simulink model "iq"  (R2021a)
settings: Solver=VariableStepAuto  StartTime=0.0  StopTime=0.2  FixedStep=1/150000  MaxStep=1e-6
undefined symbols (not defined in the file): in, ou
libraries: neural x55, spsMosfetLib x12, simulink x5, pid_lib x3, spsFirstOrderFilterLib x2, spsPermanentMagnetSynchronousMachineLib x2, spsCurrentMeasurementLib x2, spsDCVoltageSourceLib x2, spsThreePhaseVIMeasurementLib x2, spsabctoAlphaBetaZeroLib x2, spsabctodq0Lib x2, spsSVPWMGenerator2LevelLib x1
(part 3 of 5)

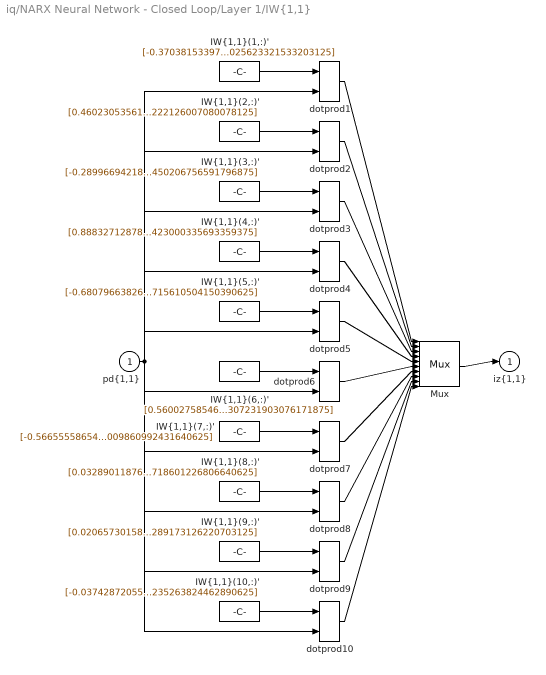
== system iq/NARX Neural Network - Closed Loop/Layer 1/IW{1,1} ==
  "pd{1,1}" : Inport  PortDimensions=40  SampleTime=1e-05
      mask Display: e = 0.06;c1 = [120 230 180]/255;c2 = ([120 230 180]+0)/(256+128);c3 = ([120 230 180]+128)/(256+128);patch([0 1 1 0],[0 0 1 1],c1);patch([0 1 1 1-e 1-e 0+e],[0 0 1 1-e 0+e 0+e],c2);patch([0 0 1 1-e 0+e 0+e],[0 1 1 1-e 1-e 0+e],c3);plot([0 1 1 0 0],[0 0 1 1 0]);
  "IW{1,1}(1,:)'" : Constant  Value=[-0.370381533971269993887887039818451739847660064697265625;-0.60836575089238376090605697754654102027416229248046875;-0.409154141847963559452949766637175343930721282958984375;-0.41099431863818447485670048990868963301181793212890625;0.582923557528958635742810656665824353694915771484375;0.48663433989662652212615512326010502874851226806640625;-0.36467940418610844677260729440604336559772491455078125;-0.357974175848268572064370118823717348277568817138671875;-0.05688146982302262621988830915142898447811603546142578125;0.27270848568918271137562214789795689284801483154296875;-0.278331288705670865102348443542723543941974639892578125;-0.297309238840328504682730681452085264027118682861328125;0.01329069212345795371332801693142755539156496524810791015625;0.147003708510372421702783185537555254995822906494140625;-0.18739990347048396390761126895085908472537994384765625;-0.2149201060465101564833645397811778821051120758056640625;-0.0917872157463859028592167987881111912429332733154296875;0.0035005746246020616983807283162377643748186528682708740234375;-0.08414655753051160369526684235097491182386875152587890625;-0.11492868974622892641601623608949012123048305511474609375;-0.06482294244093385338079116309017990715801715850830078125;-0.019538025462217778471796236772206611931324005126953125;0.0219420954523434526273195643852886860258877277374267578125;-0.000970026128533838329949523515693954323069192469120025634765625;0.1843367033017555833840361856346135027706623077392578125;0.130725146693732197089587998561910353600978851318359375;0.1154576707265280166581078447052277624607086181640625;0.12260015593334148975568353989729075692594051361083984375;-0.01254060663158583326104444921611502650193870067596435546875;0.10900370676490478416553742135874927043914794921875;0.222478076142917646773611295429873280227184295654296875;0.25070616152984681601623151436797343194484710693359375;-0.018515784184349119712020836914234678260982036590576171875;0.1284041153197590101608938084609690122306346893310546875;0.3337859120951376379338171318522654473781585693359375;0.383812488121198780444132125921896658837795257568359375;0.0961455234077264464520595765861799009144306182861328125;0.0307125609366359804408563860533831757493317127227783203125;0.446930741411597498569108211086131632328033447265625;0.5295339428349887800351325495284982025623321533203125]
      mask Display: e = 0.06;c1 = [120 150 230]/255;c2 = ([120 150 230]+0)/383;c3 = ([120 150 230]+128)/383;patch([0 1 1 0],[0 0 1 1],c1);patch([0 1 1 1-e 1-e 0+e],[0 0 1 1-e 0+e 0+e],c2);patch([0 0 1 1-e 0+e 0+e],[0 1 1 1-e 1-e 0+e],c3);plot([0 1 1 0 0],[0 0 1 1 0]);disp('Weights');
  "IW{1,1}(10,:)'" : Constant  Value=[-0.0374287205513150755820106496685184538364410400390625;0.70434564124573639798398971834103576838970184326171875;0.7522702909022649375714308916940353810787200927734375;-0.01261093693687474932840775210252104443497955799102783203125;-0.16170253340786666651496261692955158650875091552734375;-0.474734846451803138567271389547386206686496734619140625;0.58439215063359239987761384327313862740993499755859375;-0.023452774793525442420527582498834817670285701751708984375;-0.051992213555422862880650569650242687202990055084228515625;-0.402207742424022074434475371162989176809787750244140625;0.42010037354778428930757172565790824592113494873046875;-0.0264409316169393060480530266431742347776889801025390625;-0.1008865583285370182142770545397070236504077911376953125;-0.07089440261923037056579488535135169513523578643798828125;0.25870929446493751147073680840549059212207794189453125;-0.03930245328464300469395453774268389679491519927978515625;-0.15201157241618290516527167710592038929462432861328125;0.0679762667751536431293146733878529630601406097412109375;0.10520308939002430415055044932159944437444210052490234375;-0.0519526257417461945209424811764620244503021240234375;0.112774459926445358437518962091417051851749420166015625;0.12084052506689790806859718941268511116504669189453125;-0.052530615658511088661430932233997737057507038116455078125;-0.05120989834213336699964003173590754158794879913330078125;-0.12787210870842657950419152257381938397884368896484375;-0.078859476464717970234374888605088926851749420166015625;-0.182759134971150760673452850824105553328990936279296875;-0.037707706527031710497244176849562791176140308380126953125;-0.1480260727570686107856801072557573206722736358642578125;-0.0898293705578910028908268259328906424343585968017578125;-0.30135726108675431333949745749123394489288330078125;-0.0159454355043238717171139029460391611792147159576416015625;-0.1729662225865224167709044422736042179167270660400390625;-0.1563023964206002036636533603086718358099460601806640625;-0.405696085122499605635226771482848562300205230712890625;0.015662463760211853269765924778766930103302001953125;-0.06488524778837374828999173814736423082649707794189453125;0.08054078478975036647913299248102703131735324859619140625;-0.51152581330454705010879479232244193553924560546875;0.04378511372238913512688895934843458235263824462890625]
      mask Display: e = 0.06;c1 = [120 150 230]/255;c2 = ([120 150 230]+0)/383;c3 = ([120 150 230]+128)/383;patch([0 1 1 0],[0 0 1 1],c1);patch([0 1 1 1-e 1-e 0+e],[0 0 1 1-e 0+e 0+e],c2);patch([0 0 1 1-e 0+e 0+e],[0 1 1 1-e 1-e 0+e],c3);plot([0 1 1 0 0],[0 0 1 1 0]);disp('Weights');
  "IW{1,1}(2,:)'" : Constant  Value=[0.460230535615414770855835513430065475404262542724609375;-0.77110343400352954201792954336269758641719818115234375;-0.568625192561625691922699843416921794414520263671875;-0.919509208600904681674137464142404496669769287109375;-0.39640401774455680250497380257002077996730804443359375;0.7419835566523342862410572706721723079681396484375;-0.381755551532974302109124664639239199459552764892578125;-0.7087456477505529317539867406594567000865936279296875;-0.17918201870643091222490284053492359817028045654296875;0.267758509192989324620981506086536683142185211181640625;-0.2141562734063510997639667721159639768302440643310546875;-0.485468237640969968449411453548236750066280364990234375;0.073912236857971047587767543518566526472568511962890625;0.26681110876441505030953749155742116272449493408203125;-0.080785181060193222979393112836987711489200592041015625;-0.2730384489657227131687022847472690045833587646484375;0.09814172198222148590929236888769082725048065185546875;-0.08909387758340860108408065798357711173593997955322265625;0.039749900469693899562884098486392758786678314208984375;-0.05800184652617428049392600541978026740252971649169921875;0.147574973016074306730871512627345509827136993408203125;0.04308671529850323367316633493828703649342060089111328125;0.130408267684685441611946998818893916904926300048828125;0.1348065234961521030587761060814955271780490875244140625;-0.035294468563225718515941053965434548445045948028564453125;0.28432752792736992741851054233848117291927337646484375;0.1983070009014270829172943422236130572855472564697265625;0.29475254405058526341321112340665422379970550537109375;-0.016915156436537744089054768892310676164925098419189453125;-0.09312823029828450061007316662653465755283832550048828125;0.251294687102783631527103125335997901856899261474609375;0.461101599635295122947553636549855582416057586669921875;-0.162608638323653076351860136128379963338375091552734375;0.408595382101353654658026925972080789506435394287109375;0.26927948437930115943572673131711781024932861328125;0.58503349618581890201340911517036147415637969970703125;0.11881198136028313372403175662839203141629695892333984375;-0.09377170413647316349337046403888962231576442718505859375;0.26127238356779469707902308073244057595729827880859375;0.732367307705452663668665991281159222126007080078125]
      mask Display: e = 0.06;c1 = [120 150 230]/255;c2 = ([120 150 230]+0)/383;c3 = ([120 150 230]+128)/383;patch([0 1 1 0],[0 0 1 1],c1);patch([0 1 1 1-e 1-e 0+e],[0 0 1 1-e 0+e 0+e],c2);patch([0 0 1 1-e 0+e 0+e],[0 1 1 1-e 1-e 0+e],c3);plot([0 1 1 0 0],[0 0 1 1 0]);disp('Weights');
  "IW{1,1}(3,:)'" : Constant  Value=[-0.28996694218490970396118200369528494775295257568359375;-0.36061124809005706826070536408224143087863922119140625;-0.54588327055422858347100145692820660769939422607421875;0.69502750072648822321497164011816494166851043701171875;0.459811052688676780153542722473503090441226959228515625;0.1707028049477272435563435237781959585845470428466796875;-0.475962609033152961313106743546086363494396209716796875;0.50984171052008553370882282251841388642787933349609375;0.234511706529854480063335131490021012723445892333984375;0.251399622546053247429398425083491019904613494873046875;-0.38718609350964694471031180000863969326019287109375;0.328125900743076515109208912690519355237483978271484375;0.1264556506991560136388130786144756712019443511962890625;-0.01224624219050504843331328430622306768782436847686767578125;-0.27533044462442202160445958725176751613616943359375;0.1713052612391705309402567536380956880748271942138671875;-0.06355666998289448421655123411255772225558757781982421875;-0.1187766752209436782461438042446388863027095794677734375;-0.140942293439800969689912335525150410830974578857421875;0.0288957975377557747809209587330769863910973072052001953125;-0.00233847930433675986472419339179396047256886959075927734375;-0.239419891462854639296864434072631411254405975341796875;0.004712953436917500203706676842330125509761273860931396484375;-0.09205753730284167712927256843613577075302600860595703125;0.1819670548171785917634935003661666996777057647705078125;-0.0966091808059215961801413641296676360070705413818359375;0.148077918500825855829816646291874349117279052734375;-0.2020726308272137450305905304048792459070682525634765625;0.1597826280045450408895391092300997115671634674072265625;0.196815159351469315396343517932109534740447998046875;0.294673707749882662909612918156199157238006591796875;-0.316357636464268232590058005371247418224811553955078125;0.207175545789949622221826075474382378160953521728515625;0.1071998566930151552956118621295900084078311920166015625;0.4530933166326089889253125875256955623626708984375;-0.4137904547532718080304903196520172059535980224609375;0.05711111836970739208396707908832468092441558837890625;-0.1318152690200748711202294316535699181258678436279296875;0.63756481727048786023459570060367695987224578857421875;-0.4928602526792349447504193449276499450206756591796875]
      mask Display: e = 0.06;c1 = [120 150 230]/255;c2 = ([120 150 230]+0)/383;c3 = ([120 150 230]+128)/383;patch([0 1 1 0],[0 0 1 1],c1);patch([0 1 1 1-e 1-e 0+e],[0 0 1 1-e 0+e 0+e],c2);patch([0 0 1 1-e 0+e 0+e],[0 1 1 1-e 1-e 0+e],c3);plot([0 1 1 0 0],[0 0 1 1 0]);disp('Weights');
  "IW{1,1}(4,:)'" : Constant  Value=[0.8883271287804135329935206755180843174457550048828125;-0.2266246970848031783152265461467322893440723419189453125;-0.22910166788953123528926880680955946445465087890625;0.28749908493158626843211322920979000627994537353515625;-0.81981555729612332061861934562330134212970733642578125;0.20787118675508831078246885226690210402011871337890625;-0.1763409013946483916424057269978220574557781219482421875;0.27718077656700879085605038198991678655147552490234375;0.02024161448438875632316324981729849241673946380615234375;0.1209494871763732992686612988109118305146694183349609375;-0.1509565348101934156854753155130310915410518646240234375;0.2651449930152385281445504006114788353443145751953125;0.14859707956358703118127095876843668520450592041015625;-0.09396137422778279291168956888213870115578174591064453125;-0.1155763432415368441308345381912658922374248504638671875;0.2386237331347563495054231452741078101098537445068359375;0.2379874614397861354309071657553431577980518341064453125;-0.0995730806320202777026651119740563444793224334716796875;-0.07522106707113328238900606947936466895043849945068359375;0.1846894102179864882717907903497689403593540191650390625;0.11519373993966443292524814978605718351900577545166015625;-0.11286677823601802550523842683105613104999065399169921875;-0.0189903346302985158444709412606243859045207500457763671875;0.09683000749972935083942360279252170585095882415771484375;-0.1161537107331131746246200009409221820533275604248046875;-0.03160337177255623242189130905899219214916229248046875;0.0553682579867200985734854157271911390125751495361328125;-0.033970334910642295545013524815658456645905971527099609375;0.256851688248085796573150219046510756015777587890625;0.01186991873420296765562209628797063487581908702850341796875;0.1205088141197200590770677308682934381067752838134765625;-0.1906875481249030723773785211960785090923309326171875;-0.11631418104128743440384141649701632559299468994140625;0.016715536125196002459336597212313790805637836456298828125;0.2128321058880657812295567055116407573223114013671875;-0.393185645921545201542102176972548477351665496826171875;0.177559845510051494965608753773267380893230438232421875;-0.05558491458485077807427643392657046206295490264892578125;0.303322518423235598650222755168215371668338775634765625;-0.6201889351752212231616567805758677423000335693359375]
      mask Display: e = 0.06;c1 = [120 150 230]/255;c2 = ([120 150 230]+0)/383;c3 = ([120 150 230]+128)/383;patch([0 1 1 0],[0 0 1 1],c1);patch([0 1 1 1-e 1-e 0+e],[0 0 1 1-e 0+e 0+e],c2);patch([0 0 1 1-e 0+e 0+e],[0 1 1 1-e 1-e 0+e],c3);plot([0 1 1 0 0],[0 0 1 1 0]);disp('Weights');
  "IW{1,1}(5,:)'" : Constant  Value=[-0.680796638261282449633426949731074273586273193359375;-0.03561815644819237014484514247669721953570842742919921875;0.279932133091922719092536908647161908447742462158203125;-0.10665009028932870283057354754419066011905670166015625;0.177122490928476150617854045776766724884510040283203125;-0.0300441026413980454001784181627954239957034587860107421875;0.272390797246529536845827124125207774341106414794921875;-0.0788301038532349396259490958982496522367000579833984375;0.14395591702314758375536030143848620355129241943359375;-0.08272953268219518374593235421343706548213958740234375;0.250887638870884555064577625671518035233020782470703125;-0.051401743765815861852974677503880229778587818145751953125;-0.0508382055521619247162590227162581868469715118408203125;0.0020392428644184861473431791267785229138098657131195068359375;0.2195027722068458031490223447690368629992008209228515625;-0.036749789443639595265533870360741275362670421600341796875;-0.08095333598490343784970235674336436204612255096435546875;0.081837485746553084720034121346543543040752410888671875;0.1704908878112386394487742791170603595674037933349609375;-0.0307251260379036057746038324012261000461876392364501953125;-0.165691611275307959516567279933951795101165771484375;-0.0303998121496753363757203914019555668346583843231201171875;0.11201190455877886587021663444829755462706089019775390625;-0.0249260492917262842238468323330380371771752834320068359375;0.107757730517212435561447136933566071093082427978515625;-0.07092323120523795487724072472701664082705974578857421875;0.0250408958506243665975699030923351529054343700408935546875;-0.01307888394968519281402752341136874747462570667266845703125;-0.052352413946635499575332772792535251937806606292724609375;-0.008876351065879702073591062116975081153213977813720703125;-0.07340890457350270070779885145384469069540500640869140625;-0.0122828677187197532472140437675989232957363128662109375;-0.195843361485351918904740387006313540041446685791015625;-0.03310442889738003657829068515638937242329120635986328125;-0.1812967948897137027142179022121126763522624969482421875;-0.0164389600359228504888875477263354696333408355712890625;-0.327171076993585552283860806710436008870601654052734375;0.00908438331547560366796556508006688090972602367401123046875;-0.301162130493396684727258616476319730281829833984375;-0.0284852552431903750795871843592976802028715610504150390625]
      mask Display: e = 0.06;c1 = [120 150 230]/255;c2 = ([120 150 230]+0)/383;c3 = ([120 150 230]+128)/383;patch([0 1 1 0],[0 0 1 1],c1);patch([0 1 1 1-e 1-e 0+e],[0 0 1 1-e 0+e 0+e],c2);patch([0 0 1 1-e 0+e 0+e],[0 1 1 1-e 1-e 0+e],c3);plot([0 1 1 0 0],[0 0 1 1 0]);disp('Weights');
  "IW{1,1}(6,:)'" : Constant  Value=[0.5600275854677396747405282440013252198696136474609375;-0.06305175678744877332260188040891080163419246673583984375;0.40078303615261134940084275513072498142719268798828125;-0.692925615025965502269400531076826155185699462890625;-0.70120989886185103312499222738551907241344451904296875;0.101836516784308439564910031549516133964061737060546875;0.30569148245084132309301594432326965034008026123046875;-0.5069883147844633786149870502413250505924224853515625;0.04052940146582036107236746147464145906269550323486328125;-0.0638410019530132044618397912927321158349514007568359375;0.1935674074952358214574132944107986986637115478515625;-0.309998667122441673438260067996452562510967254638671875;-0.17849242641992690838748103487887419760227203369140625;0.10199276436233824238986045429555815644562244415283203125;0.098837515056082680953153385416953824460506439208984375;-0.1458748174317745782690991518393275327980518341064453125;-0.0208091413971462323162509022722588269971311092376708984375;0.06562148261369567248113554569499683566391468048095703125;0.008785509341242996039778034855771693401038646697998046875;0.004860584086910021105187862389129804796539247035980224609375;-0.017611275602437449772086353050326579250395298004150390625;0.07382029502171290336054454428449389524757862091064453125;-0.06992535386558691723468683676401269622147083282470703125;0.1339735017182300536031647197887650690972805023193359375;-0.2405850388919813787058643583804951049387454986572265625;0.12204188980898265926011703186304657720029354095458984375;-0.1272594208964332451738954432585160247981548309326171875;0.23078664969600470868726915796287357807159423828125;0.0971691048765602471970481701646349392831325531005859375;-0.11153337214839438573665830745085258968174457550048828125;-0.1817652942936347215674430799481342546641826629638671875;0.3226546000737464670038434633170254528522491455078125;-0.04269885039361918932510064905727631412446498870849609375;0.0691585842665914662941162305287434719502925872802734375;-0.221872440805359671944785304731340147554874420166015625;0.371059616443993933732059531394043006002902984619140625;-0.12310303115093119974421398410413530655205249786376953125;0.0030479467126750541157431673155997486901469528675079345703125;-0.24382769564521000749124368667253293097019195556640625;0.387797992595797225146014852725784294307231903076171875]
      mask Display: e = 0.06;c1 = [120 150 230]/255;c2 = ([120 150 230]+0)/383;c3 = ([120 150 230]+128)/383;patch([0 1 1 0],[0 0 1 1],c1);patch([0 1 1 1-e 1-e 0+e],[0 0 1 1-e 0+e 0+e],c2);patch([0 0 1 1-e 0+e 0+e],[0 1 1 1-e 1-e 0+e],c3);plot([0 1 1 0 0],[0 0 1 1 0]);disp('Weights');
  "IW{1,1}(7,:)'" : Constant  Value=[-0.56655558654103621574193994092638604342937469482421875;-0.398673686871792665176172931751352734863758087158203125;0.122259597258337848746378995201666839420795440673828125;0.51933566122342711413040206025470979511737823486328125;0.43939288349859306759270793918403796851634979248046875;0.5123719836735494137514024259871803224086761474609375;0.0711592910026745129048464377774507738649845123291015625;0.39403987044743871148710923080216161906719207763671875;0.04577065888191818310293257354715024121105670928955078125;-0.2419016469493377174959647391006001271307468414306640625;0.059322270944772881318129975625197403132915496826171875;0.297835589603741068831510574455023743212223052978515625;0.048264046454816390829822836394669138826429843902587890625;-0.142596881111394180319251745459041558206081390380859375;0.041348530547222171749321972811230807565152645111083984375;0.196466143790522795864461613746243529021739959716796875;0.00379058416686700420938915812030245433561503887176513671875;-0.1295052996036833992121728442725725471973419189453125;0.02039056123350617422129715805567684583365917205810546875;0.09166785703957426589827406360200257040560245513916015625;-0.05998331728420390474010304160401574335992336273193359375;-0.0499504038108496140058178980325465090572834014892578125;-0.004612829733083904926171925353628466837108135223388671875;-0.022829417619203706824038135891896672546863555908203125;0.10272523640724039173388604240244603715837001800537109375;0.057497579157354893053533118063569418154656887054443359375;-0.04543915315477524419218724460733938030898571014404296875;-0.14405175437682526951022055072826333343982696533203125;-0.119630288848869115181372535516857169568538665771484375;-0.24153120449403286951195468645892105996608734130859375;-0.0717540855639570429591600486673996783792972564697265625;-0.26434900172423103636987207210040651261806488037109375;0.11680165056984685711949367714623804204165935516357421875;-0.015242016961960182241941907932414324022829532623291015625;-0.12090178545372003149349637851628358475863933563232421875;-0.401554755884511560548588704477879218757152557373046875;-0.06705789660066063806453939832863397896289825439453125;-0.037242704896520380242197489906175178475677967071533203125;-0.1659638091937474524417694965450209565460681915283203125;-0.5571105664409119473390319399186410009860992431640625]
      mask Display: e = 0.06;c1 = [120 150 230]/255;c2 = ([120 150 230]+0)/383;c3 = ([120 150 230]+128)/383;patch([0 1 1 0],[0 0 1 1],c1);patch([0 1 1 1-e 1-e 0+e],[0 0 1 1-e 0+e 0+e],c2);patch([0 0 1 1-e 0+e 0+e],[0 1 1 1-e 1-e 0+e],c3);plot([0 1 1 0 0],[0 0 1 1 0]);disp('Weights');
  "IW{1,1}(8,:)'" : Constant  Value=[0.032890118763431432091781658755280659534037113189697265625;0.322573939495580608305402847690857015550136566162109375;-0.2020097790587629671410496712269377894699573516845703125;0.120414542774892663334895814841729588806629180908203125;0.481335601188250639115295825831708498299121856689453125;-0.08733088898441565550712084586848504841327667236328125;-0.170409257637735789270294617381296120584011077880859375;0.1204733773267963325981355637850356288254261016845703125;0.1929216806619530599764544831487000919878482818603515625;-0.118934269814700510625726792568457312881946563720703125;-0.1320561398595039570569298348345910198986530303955078125;0.113182030753253892729759400026523508131504058837890625;-0.09047481631882929586918606901235762052237987518310546875;-0.036344259941230895594177496832344331778585910797119140625;-0.0896966613953761038313672315780422650277614593505859375;0.09213446476664077788854001482832245528697967529296875;-0.13858299956713160394627948335255496203899383544921875;0.0150460193910525071026018650854894076474010944366455078125;-0.05402245583233598880124048946527182124555110931396484375;0.06540083056512678572058661075061536394059658050537109375;-0.129446864723562315990790239084162749350070953369140625;0.04664097095482293287016517524534719996154308319091796875;-0.0266863686150647823336345965117288869805634021759033203125;0.03499045828118012291252370005167904309928417205810546875;0.06957822701625983319306811836213455535471439361572265625;-0.000369494646568858183151295992985296834376640617847442626953125;-0.01470178937249874175086095107189976260997354984283447265625;0.0103856813377103847362281641153458622284233570098876953125;0.06895768218806731797432263419977971352636814117431640625;-0.02115769194954782161932627104761195369064807891845703125;-0.00923542554835122576906147884301390149630606174468994140625;-0.01502525587422143781013428309734081267379224300384521484375;0.1786809470977023528437399590984568931162357330322265625;-0.0199048070138533005069003678499939269386231899261474609375;-0.01654293491199494703369765602474217303097248077392578125;-0.039041310953076981127285449701957986690104007720947265625;0.400409863135611943096847653578151948750019073486328125;0.011681447993090454673392741824500262737274169921875;-0.043070406675709056731893298319846508093178272247314453125;-0.05958230402351040455588560007527121342718601226806640625]
      mask Display: e = 0.06;c1 = [120 150 230]/255;c2 = ([120 150 230]+0)/383;c3 = ([120 150 230]+128)/383;patch([0 1 1 0],[0 0 1 1],c1);patch([0 1 1 1-e 1-e 0+e],[0 0 1 1-e 0+e 0+e],c2);patch([0 0 1 1-e 0+e 0+e],[0 1 1 1-e 1-e 0+e],c3);plot([0 1 1 0 0],[0 0 1 1 0]);disp('Weights');
  "IW{1,1}(9,:)'" : Constant  Value=[0.0206573015818778855934301219576809671707451343536376953125;-0.5127945857042188748664557351730763912200927734375;0.18167984043783658165693850605748593807220458984375;0.04888427657857154218223882935490109957754611968994140625;-0.034928672254442759415038466386249638162553310394287109375;0.612016796760034953450713146594353020191192626953125;0.15951797292033376152176060713827610015869140625;0.0964910574361543538213226156585733406245708465576171875;0.132653026261133621943599791848100721836090087890625;-0.183903108710759377597554475869401358067989349365234375;0.1411277505189241499028440784968552179634571075439453125;0.15699933591514092512397837708704173564910888671875;-0.07471396464858927333185789620983996428549289703369140625;-0.08647891344068991958948799947393126785755157470703125;0.11800727913563906212868204193000565283000469207763671875;0.1723425390568689985482109250369830988347530364990234375;-0.116902071527464179734323579396004788577556610107421875;-0.054687890350883693046935007942010997794568538665771484375;0.0848725296780153681819314215317717753350734710693359375;0.1507662499010935797105759093028609640896320343017578125;-0.0263068354601329081055016700929627404548227787017822265625;-0.07978144317701051091429320649695000611245632171630859375;0.037380390586757843152110325490866671316325664520263671875;0.098847497533154804472133037052117288112640380859375;-0.09377165532459739993864644702625810168683528900146484375;0.074862603076867706430874704892630688846111297607421875;-0.023608817789773091366800628065902856178581714630126953125;0.003626695723370344619229665994453171151690185070037841796875;0.101633913513693940888771294339676387608051300048828125;-0.159021970451373173549569628448807634413242340087890625;-0.09929257206222498466363646230092854239046573638916015625;-0.10586037280174027952472926017435383982956409454345703125;0.03260980890892317685114676351076923310756683349609375;-0.111766963043459954807445910773822106420993804931640625;-0.1869791095185237284059809326208778657019138336181640625;-0.249574691397737635778497633509687148034572601318359375;-0.06307633222916309012617830376257188618183135986328125;0.0280907974422784818824272434767408412881195545196533203125;-0.288493529682975646810660919072688557207584381103515625;-0.431998237128097539727633602524292655289173126220703125]
      mask Display: e = 0.06;c1 = [120 150 230]/255;c2 = ([120 150 230]+0)/383;c3 = ([120 150 230]+128)/383;patch([0 1 1 0],[0 0 1 1],c1);patch([0 1 1 1-e 1-e 0+e],[0 0 1 1-e 0+e 0+e],c2);patch([0 0 1 1-e 0+e 0+e],[0 1 1 1-e 1-e 0+e],c3);plot([0 1 1 0 0],[0 0 1 1 0]);disp('Weights');
  Mux : Mux  Inputs=10
      mask Display: e = 0.06;c1 = [120 150 230]/255;c2 = ([120 150 230]+0)/383;c3 = ([120 150 230]+128)/383;patch([0 1 1 0],[0 0 1 1],c1);patch([0 1 1 1-e 1-e 0+e],[0 0 1 1-e 0+e 0+e],c2);patch([0 0 1 1-e 0+e 0+e],[0 1 1 1-e 1-e 0+e],c3);plot([0 1 1 0 0],[0 0 1 1 0]);disp('Mux');
  dotprod{1..10} (10 alike) : neural/Weight Functions/dotprod
  "iz{1,1}" : Outport
      mask Display: e = 0.06;c1 = [120 230 180]/255;c2 = ([120 230 180]+0)/(256+128);c3 = ([120 230 180]+128)/(256+128);patch([0 1 1 0],[0 0 1 1],c1);patch([0 1 1 1-e 1-e 0+e],[0 0 1 1-e 0+e 0+e],c2);patch([0 0 1 1-e 0+e 0+e],[0 1 1 1-e 1-e 0+e],c3);plot([0 1 1 0 0],[0 0 1 1 0]);
  wires:
  "IW{1,1}(1,:)'"/1 -> dotprod1/1
  "pd{1,1}"/1 -> dotprod1/2, dotprod2/2, dotprod3/2, dotprod4/2, dotprod5/2, dotprod6/2, dotprod7/2, dotprod8/2, dotprod9/2, dotprod10/2
  dotprod1/1 -> Mux/1
  "IW{1,1}(2,:)'"/1 -> dotprod2/1
  dotprod2/1 -> Mux/2
  "IW{1,1}(3,:)'"/1 -> dotprod3/1
  dotprod3/1 -> Mux/3
  "IW{1,1}(4,:)'"/1 -> dotprod4/1
  dotprod4/1 -> Mux/4
  "IW{1,1}(5,:)'"/1 -> dotprod5/1
  dotprod5/1 -> Mux/5
  "IW{1,1}(6,:)'"/1 -> dotprod6/1
  dotprod6/1 -> Mux/6
  "IW{1,1}(7,:)'"/1 -> dotprod7/1
  dotprod7/1 -> Mux/7
  "IW{1,1}(8,:)'"/1 -> dotprod8/1
  dotprod8/1 -> Mux/8
  "IW{1,1}(9,:)'"/1 -> dotprod9/1
  dotprod9/1 -> Mux/9
  "IW{1,1}(10,:)'"/1 -> dotprod10/1
  dotprod10/1 -> Mux/10
  Mux/1 -> "iz{1,1}"/1

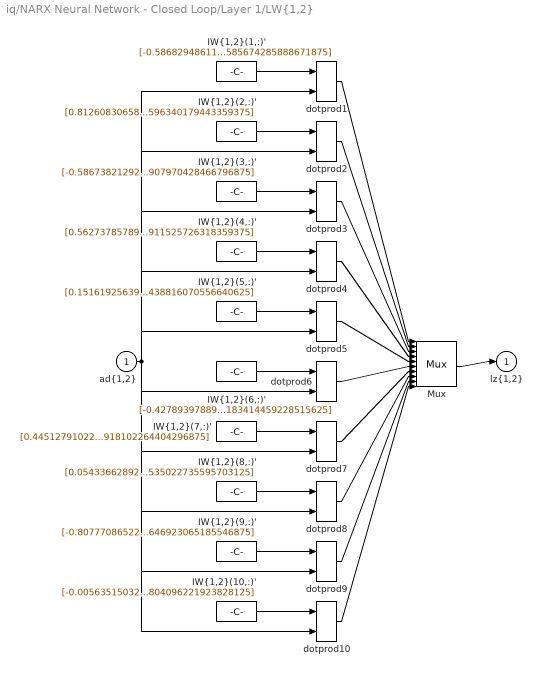
== system iq/NARX Neural Network - Closed Loop/Layer 1/LW{1,2} ==
  "ad{1,2}" : Inport  PortDimensions=10  SampleTime=1e-05
      mask Display: e = 0.06;c1 = [120 230 180]/255;c2 = ([120 230 180]+0)/(256+128);c3 = ([120 230 180]+128)/(256+128);patch([0 1 1 0],[0 0 1 1],c1);patch([0 1 1 1-e 1-e 0+e],[0 0 1 1-e 0+e 0+e],c2);patch([0 0 1 1-e 0+e 0+e],[0 1 1 1-e 1-e 0+e],c3);plot([0 1 1 0 0],[0 0 1 1 0]);
  "IW{1,2}(1,:)'" : Constant  Value=[-0.5868294861145617602460333728231489658355712890625;0.1021095008317064178893218695520772598683834075927734375;0.2603331728501079300741594124701805412769317626953125;0.288493037192464163442906510681496001780033111572265625;-0.09651029411370827537641758908648625947535037994384765625;-0.060145459247466663554870791585926781408488750457763671875;-0.08361291231078023244993602247632225044071674346923828125;0.05519399626581704410011042227779398672282695770263671875;0.11469213550091751641080151102869422174990177154541015625;-0.1602841044363691735963328710568021051585674285888671875]
      mask Display: e = 0.06;c1 = [120 150 230]/255;c2 = ([120 150 230]+0)/383;c3 = ([120 150 230]+128)/383;patch([0 1 1 0],[0 0 1 1],c1);patch([0 1 1 1-e 1-e 0+e],[0 0 1 1-e 0+e 0+e],c2);patch([0 0 1 1-e 0+e 0+e],[0 1 1 1-e 1-e 0+e],c3);plot([0 1 1 0 0],[0 0 1 1 0]);disp('weights');
  "IW{1,2}(10,:)'" : Constant  Value=[-0.00563515032061460453827184124975246959365904331207275390625;0.2160791045301600765693450512117124162614345550537109375;-0.2251843924587682288507295425006304867565631866455078125;-0.2263499968643012671964953597125713713467121124267578125;-0.0136193057826310658098289962936178199015557765960693359375;0.11016037847535209426297342361067421734333038330078125;-0.0596202034770476896330393401512992568314075469970703125;-0.025467200926077300515704138206274365074932575225830078125;0.29786664160487974495339358327328227460384368896484375;0.447752867857204694956863022525794804096221923828125]
      mask Display: e = 0.06;c1 = [120 150 230]/255;c2 = ([120 150 230]+0)/383;c3 = ([120 150 230]+128)/383;patch([0 1 1 0],[0 0 1 1],c1);patch([0 1 1 1-e 1-e 0+e],[0 0 1 1-e 0+e 0+e],c2);patch([0 0 1 1-e 0+e 0+e],[0 1 1 1-e 1-e 0+e],c3);plot([0 1 1 0 0],[0 0 1 1 0]);disp('weights');
  "IW{1,2}(2,:)'" : Constant  Value=[0.8126083065834464047583196588675491511821746826171875;-0.30999285881879501403091126121580600738525390625;-0.224119088577214464752529465840780176222324371337890625;-0.04911418181406544680722703333231038413941860198974609375;0.183795724312708685932449270694633014500141143798828125;-0.12059023823339166947565814780318760313093662261962890625;-0.08164430973522228407457390630952431820333003997802734375;0.045002408594429076094112218697773641906678676605224609375;0.1418552370000567552921211245120503008365631103515625;-0.10802203298773947748312451722085825167596340179443359375]
      mask Display: e = 0.06;c1 = [120 150 230]/255;c2 = ([120 150 230]+0)/383;c3 = ([120 150 230]+128)/383;patch([0 1 1 0],[0 0 1 1],c1);patch([0 1 1 1-e 1-e 0+e],[0 0 1 1-e 0+e 0+e],c2);patch([0 0 1 1-e 0+e 0+e],[0 1 1 1-e 1-e 0+e],c3);plot([0 1 1 0 0],[0 0 1 1 0]);disp('weights');
  "IW{1,2}(3,:)'" : Constant  Value=[-0.58673821292252770209785239785560406744480133056640625;-0.1659897726468064771410126923001371324062347412109375;0.0786947122987838587615527785601443611085414886474609375;0.354848597221148531755119392983033321797847747802734375;0.107478086904293002046273386440589092671871185302734375;0.2400276728675252713163246198746492154896259307861328125;0.000187128674300308787438462676533390549593605101108551025390625;-0.179224755384559342186179264899692498147487640380859375;-0.22230268154897192545149664510972797870635986328125;-0.1752689177342332260689516942875343374907970428466796875]
      mask Display: e = 0.06;c1 = [120 150 230]/255;c2 = ([120 150 230]+0)/383;c3 = ([120 150 230]+128)/383;patch([0 1 1 0],[0 0 1 1],c1);patch([0 1 1 1-e 1-e 0+e],[0 0 1 1-e 0+e 0+e],c2);patch([0 0 1 1-e 0+e 0+e],[0 1 1 1-e 1-e 0+e],c3);plot([0 1 1 0 0],[0 0 1 1 0]);disp('weights');
  "IW{1,2}(4,:)'" : Constant  Value=[0.56273785789506203247611892948043532669544219970703125;-0.311912916491800473739459675925900228321552276611328125;-0.21174510741117991141635457097436301410198211669921875;-0.05841110514993876068334799356307485140860080718994140625;0.03523980144411063830656161144361249171197414398193359375;-0.077203252208415451551815067432471551001071929931640625;0.0810557330681056231735936989934998564422130584716796875;0.01302129125511275638260588749517410178668797016143798828125;0.00975201502454749354076302125804431852884590625762939453125;-0.222159547481124375334360365741304121911525726318359375]
      mask Display: e = 0.06;c1 = [120 150 230]/255;c2 = ([120 150 230]+0)/383;c3 = ([120 150 230]+128)/383;patch([0 1 1 0],[0 0 1 1],c1);patch([0 1 1 1-e 1-e 0+e],[0 0 1 1-e 0+e 0+e],c2);patch([0 0 1 1-e 0+e 0+e],[0 1 1 1-e 1-e 0+e],c3);plot([0 1 1 0 0],[0 0 1 1 0]);disp('weights');
  "IW{1,2}(5,:)'" : Constant  Value=[0.151619256395423729344429375487379729747772216796875;-0.480073742880380904818338194672833196818828582763671875;0.08673378354405343604316414030108717270195484161376953125;0.1133253625013823928657785700124804861843585968017578125;-0.1213594980562381075994693446773453615605831146240234375;-0.005708387567627155011196204981160917668603360652923583984375;0.17292306362865372815207365420064888894557952880859375;0.17228379808317495491820636743796057999134063720703125;0.295738889040950636566407183636329136788845062255859375;0.6738474652504324868829144179471768438816070556640625]
      mask Display: e = 0.06;c1 = [120 150 230]/255;c2 = ([120 150 230]+0)/383;c3 = ([120 150 230]+128)/383;patch([0 1 1 0],[0 0 1 1],c1);patch([0 1 1 1-e 1-e 0+e],[0 0 1 1-e 0+e 0+e],c2);patch([0 0 1 1-e 0+e 0+e],[0 1 1 1-e 1-e 0+e],c3);plot([0 1 1 0 0],[0 0 1 1 0]);disp('weights');
  "IW{1,2}(6,:)'" : Constant  Value=[-0.42789397889618552284218822023831307888031005859375;0.11013459263892373674043057008020696230232715606689453125;0.19891698139755453755839198493049480020999908447265625;0.08345192280061260181600601981699583120644092559814453125;0.00598048883264744833565540460540432832203805446624755859375;0.046310583900698386317085208929711370728909969329833984375;-0.0469592133791627286409919861398520879447460174560546875;-0.0303041839648034404264276275853262632153928279876708984375;-0.0604670002286749885822558781001134775578975677490234375;0.157546426938095562864106113920570351183414459228515625]
      mask Display: e = 0.06;c1 = [120 150 230]/255;c2 = ([120 150 230]+0)/383;c3 = ([120 150 230]+128)/383;patch([0 1 1 0],[0 0 1 1],c1);patch([0 1 1 1-e 1-e 0+e],[0 0 1 1-e 0+e 0+e],c2);patch([0 0 1 1-e 0+e 0+e],[0 1 1 1-e 1-e 0+e],c3);plot([0 1 1 0 0],[0 0 1 1 0]);disp('weights');
  "IW{1,2}(7,:)'" : Constant  Value=[0.445127910224357103974313076832913793623447418212890625;-0.247557595534041607887587588265887461602687835693359375;-0.2244253138459708640795042811078019440174102783203125;-0.08160537906112201589348131847145850770175457000732421875;-0.11003906343633322595376711205972242169082164764404296875;0.003860977778824484750452850079227573587559163570404052734375;0.1785510870119984827564252327647409401834011077880859375;0.0220484374285307045682191784408132662065327167510986328125;-0.11703464723550054127354513866521301679313182830810546875;0.0260457104335039095477366544173492002300918102264404296875]
      mask Display: e = 0.06;c1 = [120 150 230]/255;c2 = ([120 150 230]+0)/383;c3 = ([120 150 230]+128)/383;patch([0 1 1 0],[0 0 1 1],c1);patch([0 1 1 1-e 1-e 0+e],[0 0 1 1-e 0+e 0+e],c2);patch([0 0 1 1-e 0+e 0+e],[0 1 1 1-e 1-e 0+e],c3);plot([0 1 1 0 0],[0 0 1 1 0]);disp('weights');
  "IW{1,2}(8,:)'" : Constant  Value=[0.05433662892764014318291998506538220681250095367431640625;-0.1233932067302145052511974654407822526991367340087890625;0.05782612783236755482629831703889067284762859344482421875;0.1472823379326128334643186690300353802740573883056640625;0.0139549500792485701994305458129019825719296932220458984375;-0.157135427747868039460854561184532940387725830078125;0.08050002289923714748898220250339363701641559600830078125;0.09215405466807646828186761922552250325679779052734375;-0.499503363182942361486738036546739749610424041748046875;-0.8852348943753949317425622211885638535022735595703125]
      mask Display: e = 0.06;c1 = [120 150 230]/255;c2 = ([120 150 230]+0)/383;c3 = ([120 150 230]+128)/383;patch([0 1 1 0],[0 0 1 1],c1);patch([0 1 1 1-e 1-e 0+e],[0 0 1 1-e 0+e 0+e],c2);patch([0 0 1 1-e 0+e 0+e],[0 1 1 1-e 1-e 0+e],c3);plot([0 1 1 0 0],[0 0 1 1 0]);disp('weights');
  "IW{1,2}(9,:)'" : Constant  Value=[-0.8077708652298214442311063976376317441463470458984375;0.476572027182772972597746274914243258535861968994140625;0.282047015603694106733456692381878383457660675048828125;-0.052386888619278461354245024494957760907709598541259765625;0.0953319099667691294275329028096166439354419708251953125;0.08405810700799436208097148437445866875350475311279296875;-0.061866509821340003039136234974648687057197093963623046875;-0.158041683289502354892164248667540960013866424560546875;0.05465509329875962996059257648084894753992557525634765625;0.12881415935854600984811213493230752646923065185546875]
      mask Display: e = 0.06;c1 = [120 150 230]/255;c2 = ([120 150 230]+0)/383;c3 = ([120 150 230]+128)/383;patch([0 1 1 0],[0 0 1 1],c1);patch([0 1 1 1-e 1-e 0+e],[0 0 1 1-e 0+e 0+e],c2);patch([0 0 1 1-e 0+e 0+e],[0 1 1 1-e 1-e 0+e],c3);plot([0 1 1 0 0],[0 0 1 1 0]);disp('weights');
  Mux : Mux  Inputs=10
      mask Display: e = 0.06;c1 = [120 150 230]/255;c2 = ([120 150 230]+0)/383;c3 = ([120 150 230]+128)/383;patch([0 1 1 0],[0 0 1 1],c1);patch([0 1 1 1-e 1-e 0+e],[0 0 1 1-e 0+e 0+e],c2);patch([0 0 1 1-e 0+e 0+e],[0 1 1 1-e 1-e 0+e],c3);plot([0 1 1 0 0],[0 0 1 1 0]);disp('Mux');
  dotprod{1..10} (10 alike) : neural/Weight Functions/dotprod
  "lz{1,2}" : Outport
      mask Display: e = 0.06;c1 = [120 230 180]/255;c2 = ([120 230 180]+0)/(256+128);c3 = ([120 230 180]+128)/(256+128);patch([0 1 1 0],[0 0 1 1],c1);patch([0 1 1 1-e 1-e 0+e],[0 0 1 1-e 0+e 0+e],c2);patch([0 0 1 1-e 0+e 0+e],[0 1 1 1-e 1-e 0+e],c3);plot([0 1 1 0 0],[0 0 1 1 0]);
  wires:
  "IW{1,2}(1,:)'"/1 -> dotprod1/1
  "ad{1,2}"/1 -> dotprod1/2, dotprod2/2, dotprod3/2, dotprod4/2, dotprod5/2, dotprod6/2, dotprod7/2, dotprod8/2, dotprod9/2, dotprod10/2
  dotprod1/1 -> Mux/1
  "IW{1,2}(2,:)'"/1 -> dotprod2/1
  dotprod2/1 -> Mux/2
  "IW{1,2}(3,:)'"/1 -> dotprod3/1
  dotprod3/1 -> Mux/3
  "IW{1,2}(4,:)'"/1 -> dotprod4/1
  dotprod4/1 -> Mux/4
  "IW{1,2}(5,:)'"/1 -> dotprod5/1
  dotprod5/1 -> Mux/5
  "IW{1,2}(6,:)'"/1 -> dotprod6/1
  dotprod6/1 -> Mux/6
  "IW{1,2}(7,:)'"/1 -> dotprod7/1
  dotprod7/1 -> Mux/7
  "IW{1,2}(8,:)'"/1 -> dotprod8/1
  dotprod8/1 -> Mux/8
  "IW{1,2}(9,:)'"/1 -> dotprod9/1
  dotprod9/1 -> Mux/9
  "IW{1,2}(10,:)'"/1 -> dotprod10/1
  dotprod10/1 -> Mux/10
  Mux/1 -> "lz{1,2}"/1

== system iq/NARX Neural Network - Closed Loop/Layer 2/Delays 1 ==
  "p{2}" : Inport  PortDimensions=10  SampleTime=1e-05
      mask Display: e = 0.06;c1 = [120 230 180]/255;c2 = ([120 230 180]+0)/(256+128);c3 = ([120 230 180]+128)/(256+128);patch([0 1 1 0],[0 0 1 1],c1);patch([0 1 1 1-e 1-e 0+e],[0 0 1 1-e 0+e 0+e],c2);patch([0 0 1 1-e 0+e 0+e],[0 1 1 1-e 1-e 0+e],c3);plot([0 1 1 0 0],[0 0 1 1 0]);
  mux : Mux  Inputs=1
      mask Display: e = 0.06;c1 = [120 150 230]/255;c2 = ([120 150 230]+0)/383;c3 = ([120 150 230]+128)/383;patch([0 1 1 0],[0 0 1 1],c1);patch([0 1 1 1-e 1-e 0+e],[0 0 1 1-e 0+e 0+e],c2);patch([0 0 1 1-e 0+e 0+e],[0 1 1 1-e 1-e 0+e],c3);plot([0 1 1 0 0],[0 0 1 1 0]);disp('Mux')
  "pd{2,1}" : Outport
      mask Display: e = 0.06;c1 = [120 230 180]/255;c2 = ([120 230 180]+0)/(256+128);c3 = ([120 230 180]+128)/(256+128);patch([0 1 1 0],[0 0 1 1],c1);patch([0 1 1 1-e 1-e 0+e],[0 0 1 1-e 0+e 0+e],c2);patch([0 0 1 1-e 0+e 0+e],[0 1 1 1-e 1-e 0+e],c3);plot([0 1 1 0 0],[0 0 1 1 0]);
  wires:
  "p{2}"/1 -> mux/1
  mux/1 -> "pd{2,1}"/1

== system iq/NARX Neural Network - Closed Loop/Layer 2/LW{2,1} ==
  "ad{2,1}" : Inport  PortDimensions=10  SampleTime=1e-05
      mask Display: e = 0.06;c1 = [120 230 180]/255;c2 = ([120 230 180]+0)/(256+128);c3 = ([120 230 180]+128)/(256+128);patch([0 1 1 0],[0 0 1 1],c1);patch([0 1 1 1-e 1-e 0+e],[0 0 1 1-e 0+e 0+e],c2);patch([0 0 1 1-e 0+e 0+e],[0 1 1 1-e 1-e 0+e],c3);plot([0 1 1 0 0],[0 0 1 1 0]);
  "IW{2,1}(1,:)'" : Constant  Value=[-2.05524265698425256942982741747982800006866455078125;1.3409636231968591335572682510246522724628448486328125;-0.57893723770738925171741584563278593122959136962890625;-1.8289517248038624774864047139999456703662872314453125;0.792065006187854248054236450116150081157684326171875;-2.5491733208835452018092837533913552761077880859375;-1.987490646566600904776578317978419363498687744140625;0.4852732218298358990438146065571345388889312744140625;2.095450614628716845544431635062210261821746826171875;-1.0648869020525772999263836027239449322223663330078125]
      mask Display: e = 0.06;c1 = [120 150 230]/255;c2 = ([120 150 230]+0)/383;c3 = ([120 150 230]+128)/383;patch([0 1 1 0],[0 0 1 1],c1);patch([0 1 1 1-e 1-e 0+e],[0 0 1 1-e 0+e 0+e],c2);patch([0 0 1 1-e 0+e 0+e],[0 1 1 1-e 1-e 0+e],c3);plot([0 1 1 0 0],[0 0 1 1 0]);disp('weights');
  Mux : Mux  Inputs=1
      mask Display: e = 0.06;c1 = [120 150 230]/255;c2 = ([120 150 230]+0)/383;c3 = ([120 150 230]+128)/383;patch([0 1 1 0],[0 0 1 1],c1);patch([0 1 1 1-e 1-e 0+e],[0 0 1 1-e 0+e 0+e],c2);patch([0 0 1 1-e 0+e 0+e],[0 1 1 1-e 1-e 0+e],c3);plot([0 1 1 0 0],[0 0 1 1 0]);disp('Mux');
  dotprod1 : neural/Weight Functions/dotprod
  "lz{2,1}" : Outport
      mask Display: e = 0.06;c1 = [120 230 180]/255;c2 = ([120 230 180]+0)/(256+128);c3 = ([120 230 180]+128)/(256+128);patch([0 1 1 0],[0 0 1 1],c1);patch([0 1 1 1-e 1-e 0+e],[0 0 1 1-e 0+e 0+e],c2);patch([0 0 1 1-e 0+e 0+e],[0 1 1 1-e 1-e 0+e],c3);plot([0 1 1 0 0],[0 0 1 1 0]);
  wires:
  "IW{2,1}(1,:)'"/1 -> dotprod1/1
  "ad{2,1}"/1 -> dotprod1/2
  dotprod1/1 -> Mux/1
  Mux/1 -> "lz{2,1}"/1

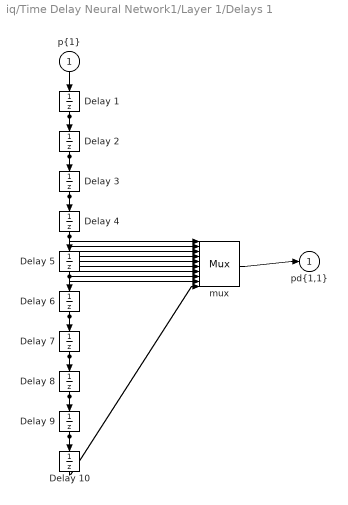
== system iq/Time Delay Neural Network1/Layer 1/Delays 1 ==
  "p{1}" : Inport  PortDimensions=4  SampleTime=1e-05
      mask Display: e = 0.06;c1 = [120 230 180]/255;c2 = ([120 230 180]+0)/(256+128);c3 = ([120 230 180]+128)/(256+128);patch([0 1 1 0],[0 0 1 1],c1);patch([0 1 1 1-e 1-e 0+e],[0 0 1 1-e 0+e 0+e],c2);patch([0 0 1 1-e 0+e 0+e],[0 1 1 1-e 1-e 0+e],c3);plot([0 1 1 0 0],[0 0 1 1 0]);
  Delay 1 : UnitDelay  InitialCondition=pi_input_1_delayed_1  SampleTime=1e-05
      mask Display: e = 0.06;c1 = [120 150 230]/255;c2 = ([120 150 230]+0)/383;c3 = ([120 150 230]+128)/383;patch([0 1 1 0],[0 0 1 1],c1);patch([0 1 1 1-e 1-e 0+e],[0 0 1 1-e 0+e 0+e],c2);patch([0 0 1 1-e 0+e 0+e],[0 1 1 1-e 1-e 0+e],c3);plot([0 1 1 0 0],[0 0 1 1 0]);disp('D')
  Delay 10 : UnitDelay  InitialCondition=pi_input_1_delayed_10  SampleTime=1e-05
      mask Display: e = 0.06;c1 = [120 150 230]/255;c2 = ([120 150 230]+0)/383;c3 = ([120 150 230]+128)/383;patch([0 1 1 0],[0 0 1 1],c1);patch([0 1 1 1-e 1-e 0+e],[0 0 1 1-e 0+e 0+e],c2);patch([0 0 1 1-e 0+e 0+e],[0 1 1 1-e 1-e 0+e],c3);plot([0 1 1 0 0],[0 0 1 1 0]);disp('D')
  Delay 2 : UnitDelay  InitialCondition=pi_input_1_delayed_2  SampleTime=1e-05
      mask Display: e = 0.06;c1 = [120 150 230]/255;c2 = ([120 150 230]+0)/383;c3 = ([120 150 230]+128)/383;patch([0 1 1 0],[0 0 1 1],c1);patch([0 1 1 1-e 1-e 0+e],[0 0 1 1-e 0+e 0+e],c2);patch([0 0 1 1-e 0+e 0+e],[0 1 1 1-e 1-e 0+e],c3);plot([0 1 1 0 0],[0 0 1 1 0]);disp('D')
  Delay 3 : UnitDelay  InitialCondition=pi_input_1_delayed_3  SampleTime=1e-05
      mask Display: e = 0.06;c1 = [120 150 230]/255;c2 = ([120 150 230]+0)/383;c3 = ([120 150 230]+128)/383;patch([0 1 1 0],[0 0 1 1],c1);patch([0 1 1 1-e 1-e 0+e],[0 0 1 1-e 0+e 0+e],c2);patch([0 0 1 1-e 0+e 0+e],[0 1 1 1-e 1-e 0+e],c3);plot([0 1 1 0 0],[0 0 1 1 0]);disp('D')
  Delay 4 : UnitDelay  InitialCondition=pi_input_1_delayed_4  SampleTime=1e-05
      mask Display: e = 0.06;c1 = [120 150 230]/255;c2 = ([120 150 230]+0)/383;c3 = ([120 150 230]+128)/383;patch([0 1 1 0],[0 0 1 1],c1);patch([0 1 1 1-e 1-e 0+e],[0 0 1 1-e 0+e 0+e],c2);patch([0 0 1 1-e 0+e 0+e],[0 1 1 1-e 1-e 0+e],c3);plot([0 1 1 0 0],[0 0 1 1 0]);disp('D')
  Delay 5 : UnitDelay  InitialCondition=pi_input_1_delayed_5  SampleTime=1e-05
      mask Display: e = 0.06;c1 = [120 150 230]/255;c2 = ([120 150 230]+0)/383;c3 = ([120 150 230]+128)/383;patch([0 1 1 0],[0 0 1 1],c1);patch([0 1 1 1-e 1-e 0+e],[0 0 1 1-e 0+e 0+e],c2);patch([0 0 1 1-e 0+e 0+e],[0 1 1 1-e 1-e 0+e],c3);plot([0 1 1 0 0],[0 0 1 1 0]);disp('D')
  Delay 6 : UnitDelay  InitialCondition=pi_input_1_delayed_6  SampleTime=1e-05
      mask Display: e = 0.06;c1 = [120 150 230]/255;c2 = ([120 150 230]+0)/383;c3 = ([120 150 230]+128)/383;patch([0 1 1 0],[0 0 1 1],c1);patch([0 1 1 1-e 1-e 0+e],[0 0 1 1-e 0+e 0+e],c2);patch([0 0 1 1-e 0+e 0+e],[0 1 1 1-e 1-e 0+e],c3);plot([0 1 1 0 0],[0 0 1 1 0]);disp('D')
  Delay 7 : UnitDelay  InitialCondition=pi_input_1_delayed_7  SampleTime=1e-05
      mask Display: e = 0.06;c1 = [120 150 230]/255;c2 = ([120 150 230]+0)/383;c3 = ([120 150 230]+128)/383;patch([0 1 1 0],[0 0 1 1],c1);patch([0 1 1 1-e 1-e 0+e],[0 0 1 1-e 0+e 0+e],c2);patch([0 0 1 1-e 0+e 0+e],[0 1 1 1-e 1-e 0+e],c3);plot([0 1 1 0 0],[0 0 1 1 0]);disp('D')
  Delay 8 : UnitDelay  InitialCondition=pi_input_1_delayed_8  SampleTime=1e-05
      mask Display: e = 0.06;c1 = [120 150 230]/255;c2 = ([120 150 230]+0)/383;c3 = ([120 150 230]+128)/383;patch([0 1 1 0],[0 0 1 1],c1);patch([0 1 1 1-e 1-e 0+e],[0 0 1 1-e 0+e 0+e],c2);patch([0 0 1 1-e 0+e 0+e],[0 1 1 1-e 1-e 0+e],c3);plot([0 1 1 0 0],[0 0 1 1 0]);disp('D')
  Delay 9 : UnitDelay  InitialCondition=pi_input_1_delayed_9  SampleTime=1e-05
      mask Display: e = 0.06;c1 = [120 150 230]/255;c2 = ([120 150 230]+0)/383;c3 = ([120 150 230]+128)/383;patch([0 1 1 0],[0 0 1 1],c1);patch([0 1 1 1-e 1-e 0+e],[0 0 1 1-e 0+e 0+e],c2);patch([0 0 1 1-e 0+e 0+e],[0 1 1 1-e 1-e 0+e],c3);plot([0 1 1 0 0],[0 0 1 1 0]);disp('D')
  mux : Mux  Inputs=10
      mask Display: e = 0.06;c1 = [120 150 230]/255;c2 = ([120 150 230]+0)/383;c3 = ([120 150 230]+128)/383;patch([0 1 1 0],[0 0 1 1],c1);patch([0 1 1 1-e 1-e 0+e],[0 0 1 1-e 0+e 0+e],c2);patch([0 0 1 1-e 0+e 0+e],[0 1 1 1-e 1-e 0+e],c3);plot([0 1 1 0 0],[0 0 1 1 0]);disp('Mux')
  "pd{1,1}" : Outport
      mask Display: e = 0.06;c1 = [120 230 180]/255;c2 = ([120 230 180]+0)/(256+128);c3 = ([120 230 180]+128)/(256+128);patch([0 1 1 0],[0 0 1 1],c1);patch([0 1 1 1-e 1-e 0+e],[0 0 1 1-e 0+e 0+e],c2);patch([0 0 1 1-e 0+e 0+e],[0 1 1 1-e 1-e 0+e],c3);plot([0 1 1 0 0],[0 0 1 1 0]);
  wires:
  "p{1}"/1 -> Delay 1/1
  Delay 1/1 -> Delay 2/1, mux/1
  Delay 2/1 -> Delay 3/1, mux/2
  Delay 3/1 -> Delay 4/1, mux/3
  Delay 4/1 -> Delay 5/1, mux/4
  Delay 5/1 -> Delay 6/1, mux/5
  Delay 6/1 -> Delay 7/1, mux/6
  Delay 7/1 -> Delay 8/1, mux/7
  Delay 8/1 -> Delay 9/1, mux/8
  Delay 9/1 -> Delay 10/1, mux/9
  Delay 10/1 -> mux/10
  mux/1 -> "pd{1,1}"/1
